simulink model "q_heli3d_semestral_project_LQR_17a"  (Simulink 8.9)
settings: Solver=ode1  StartTime=0.0  StopTime=inf  FixedStep=0.002  RelTol=1e-3  EnableMultiTasking=on
undefined symbols (not defined in the file or in its folder): elev_0, HIL, K_AMP, K_EC_E, K_EC_P, K_EC_T, qc_get_step_size, VMAX_AMP, VMAX_DAC, wcf, zetaf
libraries: quarc_library x4, simulink_extras x3
settings Model: Creator=MLevis  LastModifiedBy=obrusvit  SimulationMode=external  ExtModeTrigDuration=1000000
settings SolverCC: PositivePriorityOrder=on
settings DataIOCC: MaxDataPoints=100000
settings OptimizationCC: ExpressionDepthLimit=2147483647  InitFltsAndDblsToZero=on
settings DebuggingCC: SaveWithParameterizedLinksMsg=none  SolverPrmCheckMsg=warning
settings RTWCC: SystemTargetFile=quarc_win64.tlc  TemplateMakefile=quarc_default_tmf  Description=QUARC Win64 Target
settings STFCustomTargetCC: TargetPreCompLibLocation=C:\PROGRA~3\QUARC\lib\2017a\win64\release  ConcurrentExecutionCompliant=on  GeneratePreprocessorConditionals=Disable all  SystemTargetFile=quarc_win64.tlc
settings GRTTargetCC: TargetPreCompLibLocation=C:\PROGRA~3\QUARC\lib\2017a\win64\release  ParMdlRefBuildCompliant=off  CompOptLevelCompliant=off  MatFileLogging=off  CPPClassGenCompliant=off  UseToolchainInfoCompliant=off  ExtMode=on  ExtModeMexFile=quarc_comm

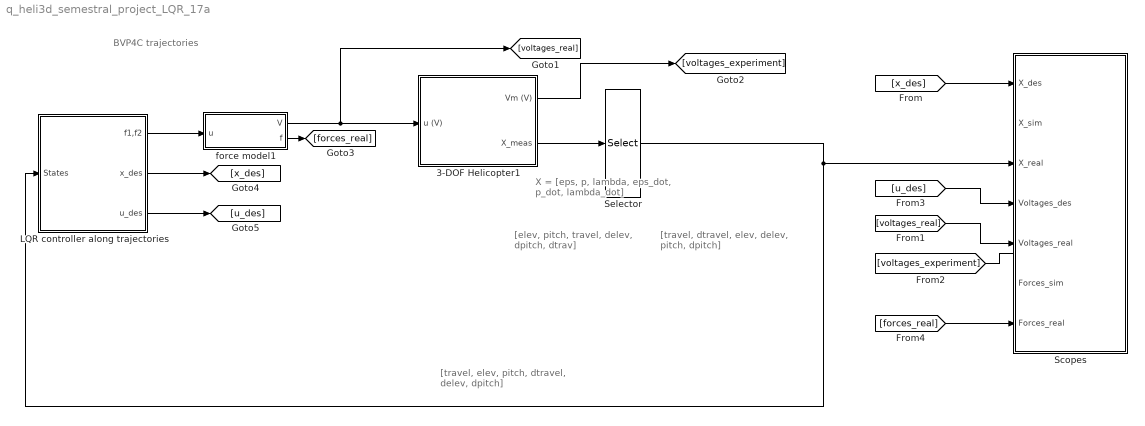
== system q_heli3d_semestral_project_LQR_17a ==
  note: BVP4C trajectories
  note: X = [eps, p, lambda, eps_dot, p_dot, lambda_dot]
  note: [elev, pitch, travel,
      | delev, dpitch, dtrav]
  note: [travel, dtravel, elev, delev, pitch, dpitch]
  note: [travel, elev, pitch,
      | dtravel, delev, dpitch]
  3-DOF Helicopter1 : Subsystem
  LQR controller along trajectories : Subsystem
  Scopes : Subsystem
  Selector : Selector  InputPortWidth=6  IndexOptions=Index vector (dialog)  Indices=[3 6 1 4 2 5]  OutputSizes=1
  force model1 : Subsystem
  wires:
  force model1/2(f) -> [forces_real]
  [forces_real] -> Scopes/7("Forces_real ")
  [voltages_real] -> Scopes/5("Voltages_real ")
  3-DOF Helicopter1/2(X_meas) -> Selector/1
  Selector/1 -> LQR controller along trajectories/1(States), Scopes/3("X_real ")
  force model1/1(V) -> [voltages_real], 3-DOF Helicopter1/1(u (V))
  3-DOF Helicopter1/1(Vm (V)) -> [voltages_experiment]
  [voltages_experiment] -> ?
  LQR controller along trajectories/1(f1,f2) -> force model1/1(u)
  LQR controller along trajectories/2(x_des) -> [x_des]
  [x_des] -> Scopes/1(X_des)
  LQR controller along trajectories/3("u_des ") -> [u_des]
  [u_des] -> Scopes/4("Voltages_des ")

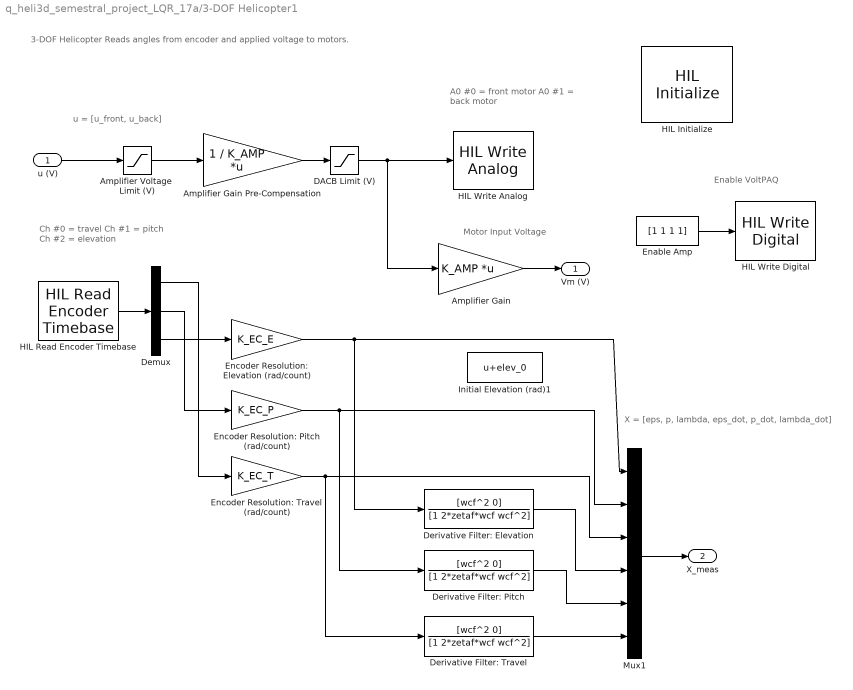
== system q_heli3d_semestral_project_LQR_17a/3-DOF Helicopter1 ==
  note: Enable VoltPAQ
  note: X = [eps, p, lambda, eps_dot, p_dot, lambda_dot]
  note: Ch #0 = travel
      | Ch #1 = pitch
      | Ch #2 = elevation
  note: 3-DOF Helicopter
      | Reads angles from encoder and applied voltage to motors.
  note: Motor Input Voltage
  note: u = [u_front, u_back]
  note: A0 #0 = front motor
      | A0 #1 = back motor
  u (V) : Inport
  Amplifier Gain : Gain  Gain=K_AMP  Multiplication=Matrix(K*u)  SaturateOnIntegerOverflow=on  OutDataTypeStr=Inherit: Same as input  ParamDataTypeStr=Inherit: Same as input
  Amplifier Gain Pre-Compensation : Gain  Gain=1 / K_AMP  Multiplication=Matrix(K*u)  SaturateOnIntegerOverflow=on  OutDataTypeStr=Inherit: Same as input  ParamDataTypeStr=Inherit: Same as input
  Amplifier Voltage  Limit (V) : Saturate  UpperLimit=VMAX_AMP  LowerLimit=-VMAX_AMP
  DACB Limit (V) : Saturate  UpperLimit=VMAX_DAC  LowerLimit=-VMAX_DAC
  Demux : Demux  Outputs=3
  Derivative Filter: Elevation : TransferFcn  Numerator=[wcf^2 0]  Denominator=[1 2*zetaf*wcf wcf^2]
  Derivative Filter: Pitch : TransferFcn  Numerator=[wcf^2 0]  Denominator=[1 2*zetaf*wcf wcf^2]
  Derivative Filter: Travel : TransferFcn  Numerator=[wcf^2 0]  Denominator=[1 2*zetaf*wcf wcf^2]
  Enable Amp : Constant  Value=[1 1 1 1]
  Encoder Resolution: Elevation (rad/count) : Gain  Gain=K_EC_E
  Encoder Resolution: Pitch (rad/count) : Gain  Gain=K_EC_P
  Encoder Resolution: Travel (rad/count) : Gain  Gain=K_EC_T
  HIL Initialize : quarc_library/Data Acquisition/Generic/Configuration/HIL Initialize  object_name=HIL-1  board_type=q8_usb  board_number=0  board_options=update_rate=normal;decimation=1  exclusive=off  active=on  hardware_clocks=[0:2]  clock_modes=[]  initial_clock_frequencies=[]  set_clock_params_at_start=off  set_clock_params_at_switch_in=off  set_clock_frequencies_at_start=off  set_clock_frequencies_at_switch_in=off  analog_input_channels=[0:7]  analog_input_configurations=[]  analog_input_maximums=10  analog_input_minimums=-10  set_analog_input_params_at_start=on  set_analog_input_params_at_switch_in=off  analog_output_channels=[0:7]  analog_output_maximums=10  analog_output_minimums=-10  initial_analog_outputs=[0]  final_analog_outputs=[0]  watchdog_analog_outputs=0  set_analog_output_params_at_start=on  set_analog_output_params_at_switch_in=off  set_analog_outputs_at_start=on  set_analog_outputs_at_switch_in=off  set_analog_outputs_at_terminate=on  set_analog_outputs_at_switch_out=off  set_analog_outputs_on_watchdog=off  digital_input_channels=[]  digital_output_channels=[]  digital_output_configuration=[]  initial_digital_outputs=[1]  final_digital_outputs=[1]  watchdog_digital_outputs=[1]  set_digital_output_params_at_start=off  set_digital_output_params_at_switch_in=off  set_digital_outputs_at_start=on  set_digital_outputs_at_switch_in=off  set_digital_outputs_at_terminate=on  set_digital_outputs_at_switch_out=off  set_digital_outputs_on_watchdog=off  encoder_channels=[0:7]  quadrature=[4]  encoder_filter_frequency=[]  initial_encoder_counts=[0]  set_encoder_params_at_start=on  set_encoder_params_at_switch_in=off  set_encoder_counts_at_start=on  set_encoder_counts_at_switch_in=off  pwm_channels=[0:7]  pwm_modes=0  pwm_frequency=99.532799999999995e6/4095  pwm_configuration=[0]  pwm_alignment=[0]  pwm_polarity=[1]  pwm_leading_deadband=[0]  pwm_trailing_deadband=[0]  initial_pwm_outputs=[0]  final_pwm_outputs=[0]  watchdog_pwm_outputs=[0]  set_pwm_params_at_start=on  set_pwm_params_at_switch_in=off  set_pwm_outputs_at_start=on  set_pwm_outputs_at_switch_in=off  set_pwm_outputs_at_terminate=on  set_pwm_outputs_at_switch_out=off  set_pwm_outputs_on_watchdog=off  other_output_channels=[]  initial_other_outputs=[]  final_other_outputs=[]  watchdog_other_outputs=[]  set_other_outputs_at_start=off  set_other_outputs_at_switch_in=off  set_other_outputs_at_terminate=off  set_other_outputs_at_switch_out=off  set_other_outputs_on_watchdog=off
  HIL Read Encoder Timebase : quarc_library/Data Acquisition/Generic/Timebases/HIL Read Encoder Timebase  object_name=HIL-1  clock=0  channels=[0:2]  samples_in_buffer=max(ceil(1/qc_get_step_size), 1)  active=on  vector_output=on  data_type_mode=Inherit via back propagation  data_type=double
  HIL Write Analog : quarc_library/Data Acquisition/Generic/Immediate I//O/HIL Write Analog  object_name=HIL-1  channels=[0,1]  sample_time=-1  active=off  vector_input=on
  HIL Write Digital : quarc_library/Data Acquisition/Generic/Immediate I//O/HIL Write Digital  object_name=HIL-1  channels=[0:3]  sample_time=-1  active=off  vector_input=on
      settings: SourceProductName=QUARC Targets
  Initial Elevation (rad)1 : Bias  Bias=elev_0
  Mux1 : Mux  Inputs=6
  Vm (V) : Outport
  X_meas : Outport  Port=2
  wires:
  Enable Amp/1 -> HIL Write Digital/1
  Encoder Resolution: Elevation (rad/count)/1 -> Mux1/1, Derivative Filter: Elevation/1
  Derivative Filter: Travel/1 -> Mux1/6
  Derivative Filter: Pitch/1 -> Mux1/5
  Derivative Filter: Elevation/1 -> Mux1/4
  Encoder Resolution: Travel (rad/count)/1 -> Derivative Filter: Travel/1, Mux1/3
  Encoder Resolution: Pitch (rad/count)/1 -> Derivative Filter: Pitch/1, Mux1/2
  Demux/2 -> Encoder Resolution: Pitch (rad/count)/1
  Demux/1 -> Encoder Resolution: Travel (rad/count)/1
  Demux/3 -> Encoder Resolution: Elevation (rad/count)/1
  DACB Limit (V)/1 -> HIL Write Analog/1, Amplifier Gain/1
  u (V)/1 -> Amplifier Voltage  Limit (V)/1
  Amplifier Gain/1 -> Vm (V)/1
  Amplifier Voltage  Limit (V)/1 -> Amplifier Gain Pre-Compensation/1
  Amplifier Gain Pre-Compensation/1 -> DACB Limit (V)/1
  Mux1/1 -> X_meas/1
  HIL Read Encoder Timebase/1 -> Demux/1

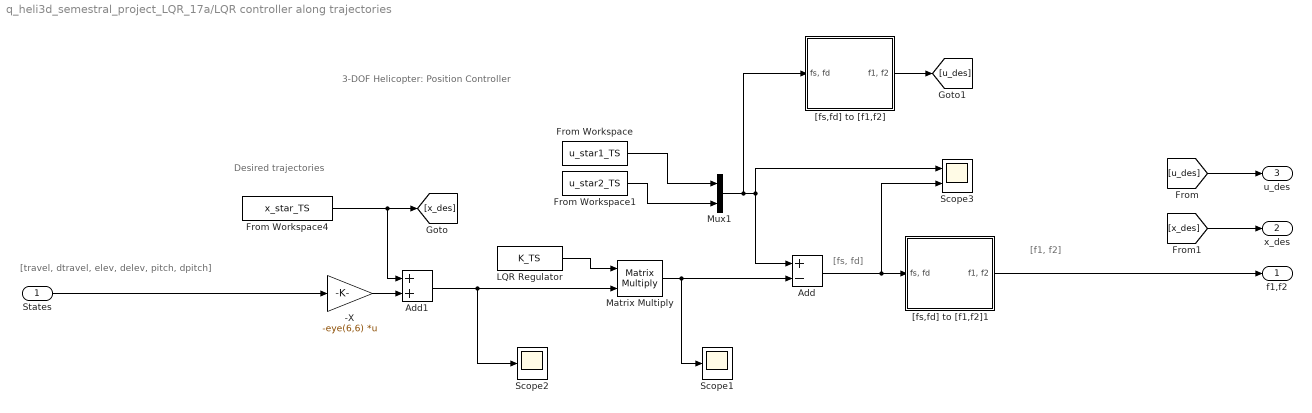
== system q_heli3d_semestral_project_LQR_17a/LQR controller along trajectories ==
  note: Desired trajectories
  note: 3-DOF Helicopter: Position Controller
  note: [travel, dtravel, elev, delev, pitch, dpitch]
  note: [fs, fd]
  note: [f1, f2]
  States : Inport
  -X : Gain  Gain=-eye(6,6)  Multiplication=Matrix(K*u)
  Add : Sum  Inputs=+-
  Add1 : Sum
  From Workspace : FromWorkspace  VariableName=u_star1_TS  SampleTime=0  Interpolate=off  OutputAfterFinalValue=Setting to zero
  From Workspace1 : FromWorkspace  VariableName=u_star2_TS  SampleTime=0  Interpolate=off  OutputAfterFinalValue=Setting to zero
  From Workspace4 : FromWorkspace  VariableName=x_star_TS  SampleTime=0  Interpolate=off  OutputAfterFinalValue=Holding final value
  LQR Regulator : FromWorkspace  VariableName=K_TS  SampleTime=0  Interpolate=off  OutputAfterFinalValue=Holding final value
  Matrix Multiply : Product  Multiplication=Matrix(*)
  Mux1 : Mux  Inputs=2
  Scope1 : Scope
  Scope2 : Scope
  Scope3 : Scope  NumInputPorts=2
  "[fs,fd] to [f1,f2]" : Subsystem
  "[fs,fd] to [f1,f2]1" : Subsystem
  f1,f2 : Outport
  x_des : Outport  Port=2
  "u_des " : Outport  Port=3
  wires:
  From Workspace4/1 -> [x_des], Add1/1
  From Workspace/1 -> Mux1/1
  -X/1 -> Add1/2
  From Workspace1/1 -> Mux1/2
  Add1/1 -> Matrix Multiply/2, Scope2/1
  Add/1 -> Scope3/2, "[fs,fd] to [f1,f2]1"/1("fs, fd")
  Matrix Multiply/1 -> Add/2, Scope1/1
  States/1 -> -X/1
  "[fs,fd] to [f1,f2]1"/1("f1, f2") -> f1,f2/1
  [x_des] -> x_des/1
  [u_des] -> "u_des "/1
  LQR Regulator/1 -> Matrix Multiply/1
  Mux1/1 -> "[fs,fd] to [f1,f2]"/1("fs, fd"), Add/1, Scope3/1
  "[fs,fd] to [f1,f2]"/1("f1, f2") -> [u_des]

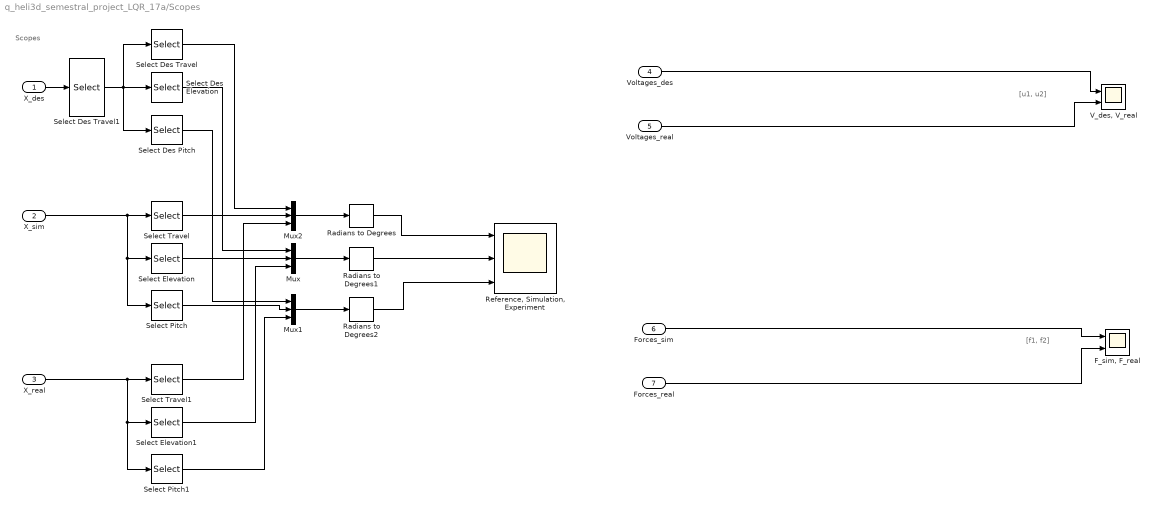
== system q_heli3d_semestral_project_LQR_17a/Scopes ==
  note: Scopes
  note: [f1, f2]
  note: [u1, u2]
  X_des : Inport
  X_sim : Inport  Port=2
  "X_real " : Inport  Port=3
  "Voltages_des " : Inport  Port=4
  "Voltages_real " : Inport  Port=5
  Forces_sim : Inport  Port=6
  "Forces_real " : Inport  Port=7
  "F_sim, F_real" : Scope  NumInputPorts=2
  Mux : Mux  Inputs=3
  Mux1 : Mux  Inputs=3
  Mux2 : Mux  Inputs=3
  Radians to Degrees : simulink_extras/Transformations/Radians to Degrees
  Radians to Degrees1 : simulink_extras/Transformations/Radians to Degrees
  Radians to Degrees2 : simulink_extras/Transformations/Radians to Degrees
  "Reference, Simulation, Experiment" : Scope  NumInputPorts=3
  Select Des Elevation : Selector  InputPortWidth=3  IndexOptions=Index vector (dialog)  Indices=2  OutputSizes=1
  Select Des Pitch : Selector  InputPortWidth=3  IndexOptions=Index vector (dialog)  Indices=3  OutputSizes=1
  Select Des Travel : Selector  InputPortWidth=3  IndexOptions=Index vector (dialog)  Indices=1  OutputSizes=1
  Select Des Travel1 : Selector  InputPortWidth=6  IndexOptions=Index vector (dialog)  Indices=[1,3,5]  OutputSizes=1
  Select Elevation : Selector  InputPortWidth=6  IndexOptions=Index vector (dialog)  Indices=3  OutputSizes=1
  Select Elevation1 : Selector  InputPortWidth=6  IndexOptions=Index vector (dialog)  Indices=3  OutputSizes=1
  Select Pitch : Selector  InputPortWidth=6  IndexOptions=Index vector (dialog)  Indices=5  OutputSizes=1
  Select Pitch1 : Selector  InputPortWidth=6  IndexOptions=Index vector (dialog)  Indices=5  OutputSizes=1
  Select Travel : Selector  InputPortWidth=6  IndexOptions=Index vector (dialog)  Indices=1  OutputSizes=1
  Select Travel1 : Selector  InputPortWidth=6  IndexOptions=Index vector (dialog)  Indices=1  OutputSizes=1
  "V_des, V_real" : Scope  NumInputPorts=2
  wires:
  Mux1/1 -> Radians to Degrees2/1
  X_sim/1 -> Select Pitch/1, Select Elevation/1, Select Travel/1
  Mux2/1 -> Radians to Degrees/1
  Select Elevation/1 -> Mux/2
  Select Pitch/1 -> Mux1/2
  Select Travel/1 -> Mux2/2
  X_des/1 -> Select Des Travel1/1
  Select Des Elevation/1 -> Mux/1
  Select Des Travel/1 -> Mux2/1
  Select Des Pitch/1 -> Mux1/1
  Mux/1 -> Radians to Degrees1/1
  "Voltages_real "/1 -> "V_des, V_real"/2
  "Forces_real "/1 -> "F_sim, F_real"/2
  "X_real "/1 -> Select Pitch1/1, Select Elevation1/1, Select Travel1/1
  Select Travel1/1 -> Mux2/3
  Select Elevation1/1 -> Mux/3
  Select Pitch1/1 -> Mux1/3
  Radians to Degrees/1 -> "Reference, Simulation, Experiment"/1
  Radians to Degrees1/1 -> "Reference, Simulation, Experiment"/2
  Radians to Degrees2/1 -> "Reference, Simulation, Experiment"/3
  "Voltages_des "/1 -> "V_des, V_real"/1
  Forces_sim/1 -> "F_sim, F_real"/1
  Select Des Travel1/1 -> Select Des Travel/1, Select Des Pitch/1, Select Des Elevation/1

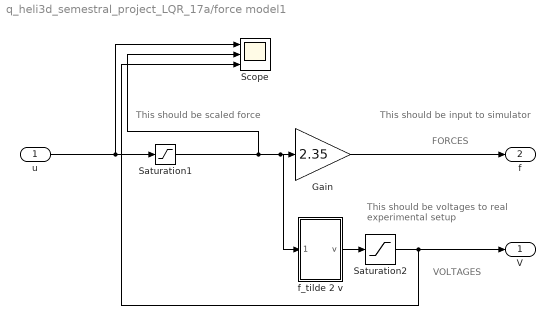
== system q_heli3d_semestral_project_LQR_17a/force model1 ==
  note: This should be voltages to
      |  real experimental setup
  note: This should be scaled force
  note: This should be input to simulator
  note: FORCES
  note: VOLTAGES
  u : Inport
  Gain : Gain  Gain=2.35
  Saturation1 : Saturate  UpperLimit=2  LowerLimit=-2
  Saturation2 : Saturate  UpperLimit=20  LowerLimit=-20
  Scope : Scope  NumInputPorts=3
  f_tilde 2 v : Subsystem
  V : Outport
  f : Outport  Port=2
  wires:
  u/1 -> Scope/1, Saturation1/1
  Gain/1 -> f/1
  Saturation1/1 -> Scope/2, f_tilde 2 v/1(f_tilde), Gain/1
  f_tilde 2 v/1(v) -> Saturation2/1
  Saturation2/1 -> Scope/3, V/1

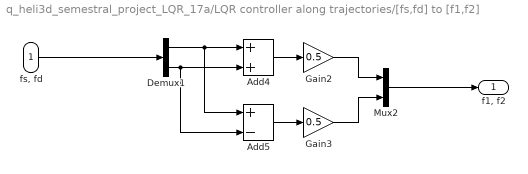
== system q_heli3d_semestral_project_LQR_17a/LQR controller along trajectories/[fs,fd] to [f1,f2] ==
  "fs, fd" : Inport
  Add4 : Sum
  Add5 : Sum  Inputs=+-
  Demux1 : Demux  Outputs=2
  Gain2 : Gain  Gain=0.5
  Gain3 : Gain  Gain=0.5
  Mux2 : Mux  Inputs=2
  "f1, f2" : Outport
  wires:
  Mux2/1 -> "f1, f2"/1
  "fs, fd"/1 -> Demux1/1
  Demux1/1 -> Add5/1, Add4/1
  Add5/1 -> Gain3/1
  Demux1/2 -> Add5/2, Add4/2
  Gain2/1 -> Mux2/1
  Add4/1 -> Gain2/1
  Gain3/1 -> Mux2/2

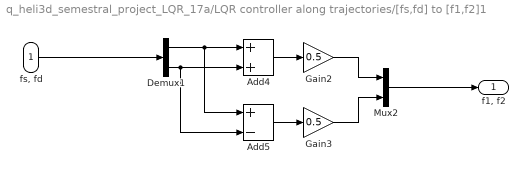
== system q_heli3d_semestral_project_LQR_17a/LQR controller along trajectories/[fs,fd] to [f1,f2]1 ==
  "fs, fd" : Inport
  Add4 : Sum
  Add5 : Sum  Inputs=+-
  Demux1 : Demux  Outputs=2
  Gain2 : Gain  Gain=0.5
  Gain3 : Gain  Gain=0.5
  Mux2 : Mux  Inputs=2
  "f1, f2" : Outport
  wires:
  Mux2/1 -> "f1, f2"/1
  "fs, fd"/1 -> Demux1/1
  Demux1/1 -> Add5/1, Add4/1
  Add5/1 -> Gain3/1
  Demux1/2 -> Add5/2, Add4/2
  Gain2/1 -> Mux2/1
  Add4/1 -> Gain2/1
  Gain3/1 -> Mux2/2

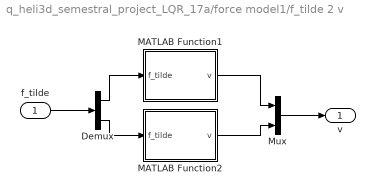
== system q_heli3d_semestral_project_LQR_17a/force model1/f_tilde 2 v ==
  f_tilde : Inport
  Demux : Demux  Outputs=2
  MATLAB Function1 : MATLAB Function  TreatAsAtomicUnit=on
  MATLAB Function2 : MATLAB Function  TreatAsAtomicUnit=on
  Mux : Mux  Inputs=2
  v : Outport
  wires:
  f_tilde/1 -> Demux/1
  Mux/1 -> v/1
  Demux/1 -> MATLAB Function1/1(f_tilde)
  Demux/2 -> MATLAB Function2/1(f_tilde)
  MATLAB Function1/1(v) -> Mux/1
  MATLAB Function2/1(v) -> Mux/2

== matlab function force model1/f_tilde 2 v/MATLAB Function1 ==
  data: f_tilde input double; v output double
function v = fcn(f_tilde)

v = scaled_force_2_voltage_new(f_tilde);

== matlab function force model1/f_tilde 2 v/MATLAB Function2 ==
  data: f_tilde input double; v output double
function v = fcn(f_tilde)

v = scaled_force_2_voltage_new(f_tilde);
